simulink model "subsystem_socrates"  (R2019b)
settings: Solver=VariableStepAuto  StartTime=0.0  StopTime=10.0  RelTol=1e-3
undefined symbols (not defined in the file or in its folder): nb_rooms, nb_step_to_fifteen_min, nb_step_to_one_h, nb_step_to_thirty_min
libraries: dspstat3 x6
settings Model: Creator=guotong  LastModifiedBy=pat
settings ModelReferenceCC: ModelReferenceNumInstancesAllowed=Single

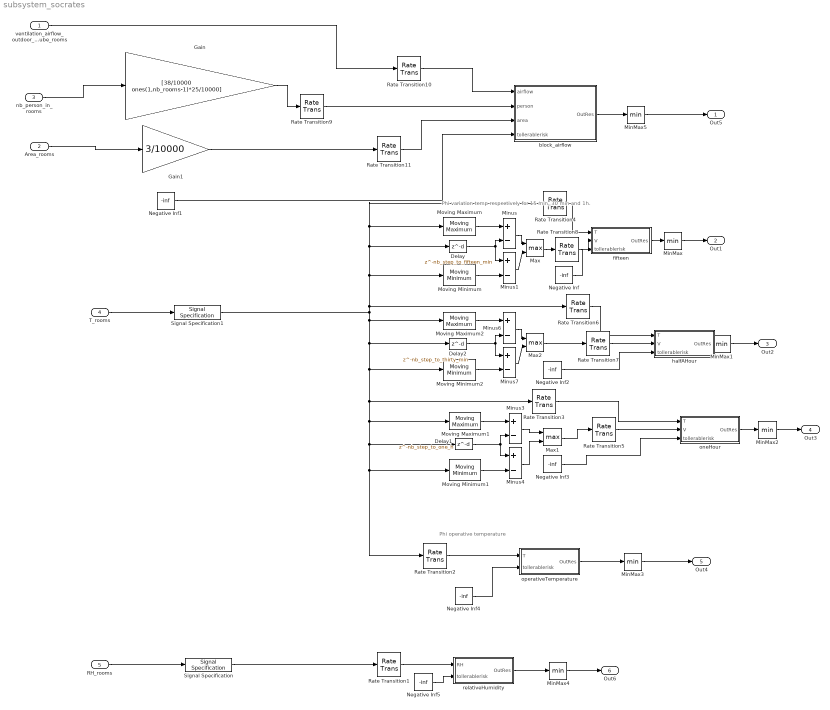
== system subsystem_socrates ==
  note: Phi operative temperature
  note: Phi variation temp respectively for 15 min, 30 min and 1h.
  ventilation_airflow_outdoor_air_mcube_rooms : Inport  PortDimensions=nb_rooms
  Area_rooms : Inport  Port=2  PortDimensions=nb_rooms
  nb_person_in_rooms : Inport  Port=3  OutDataTypeStr=double  PortDimensions=nb_rooms
  T_rooms : Inport  Port=4  PortDimensions=nb_rooms
  RH_rooms : Inport  Port=5  PortDimensions=nb_rooms
  Delay : Delay  DelayLength=nb_step_to_fifteen_min  InitialCondition=27
  Delay1 : Delay  DelayLength=nb_step_to_one_h  InitialCondition=27
  Delay2 : Delay  DelayLength=nb_step_to_thirty_min  InitialCondition=27
  Gain : Gain  Gain=[38/10000 ones(1,nb_rooms-1)*25/10000]
  Gain1 : Gain  Gain=3/10000
  Max : MinMax  Function=max  Inputs=2  ZeroCross=off
  Max1 : MinMax  Function=max  Inputs=2  ZeroCross=off
  Max2 : MinMax  Function=max  Inputs=2  ZeroCross=off
  MinMax{,1..5} (6 alike) : MinMax
  Minus{,1,3..4,6..7} (6 alike) : Sum  Inputs=+-
  Moving Maximum : dspstat3/Moving Maximum  SpecifyWindowLength=on  WindowLength=nb_step_to_fifteen_min  SimulateUsing=Code generation
      settings: SourceProductName=DSP System Toolbox  SourceProductBaseCode=DS
  Moving Maximum1 : dspstat3/Moving Maximum  SpecifyWindowLength=on  WindowLength=nb_step_to_one_h  SimulateUsing=Code generation
      settings: SourceProductName=DSP System Toolbox  SourceProductBaseCode=DS
  Moving Maximum2 : dspstat3/Moving Maximum  SpecifyWindowLength=on  WindowLength=nb_step_to_thirty_min  SimulateUsing=Code generation
      settings: SourceProductName=DSP System Toolbox  SourceProductBaseCode=DS
  Moving Minimum : dspstat3/Moving Minimum  SpecifyWindowLength=on  WindowLength=nb_step_to_fifteen_min  SimulateUsing=Code generation
      settings: SourceProductName=DSP System Toolbox  SourceProductBaseCode=DS
  Moving Minimum1 : dspstat3/Moving Minimum  SpecifyWindowLength=on  WindowLength=nb_step_to_one_h  SimulateUsing=Code generation
      settings: SourceProductName=DSP System Toolbox  SourceProductBaseCode=DS
  Moving Minimum2 : dspstat3/Moving Minimum  SpecifyWindowLength=on  WindowLength=nb_step_to_thirty_min  SimulateUsing=Code generation
      settings: SourceProductName=DSP System Toolbox  SourceProductBaseCode=DS
  Negative Inf{,1..5} (6 alike) : Constant  Value=-inf  OutDataTypeStr=Inherit: Inherit via back propagation
  Rate Transition{1..11} (11 alike) : RateTransition  OutPortSampleTime=rate
  Signal Specification : SignalSpecification  OutMin=-0.25  OutMax=1.25  Dimensions=nb_rooms
  Signal Specification1 : SignalSpecification  OutMin=-100  OutMax=100  Dimensions=nb_rooms
  block_airflow : Subsystem
  fifteen : Subsystem
  halfAHour : Subsystem
  oneHour : Subsystem
  operativeTemperature : Subsystem
  relativeHumidity : Subsystem
  Out5 : Outport
  Out1 : Outport  Port=2
  Out2 : Outport  Port=3
  Out3 : Outport  Port=4
  Out4 : Outport  Port=5
  Out6 : Outport  Port=6
  wires:
  nb_person_in_rooms/1 -> Gain/1
  Gain/1 -> Rate Transition9/1
  ventilation_airflow_outdoor_air_mcube_rooms/1 -> Rate Transition10/1
  Gain1/1 -> Rate Transition11/1
  Area_rooms/1 -> Gain1/1
  Delay2/1 -> Minus6/2, Minus7/1
  Moving Minimum1/1 -> Minus4/2
  Signal Specification1/1 -> Rate Transition2/1, Moving Minimum1/1, Delay1/1, Moving Maximum1/1, Rate Transition3/1, Moving Minimum2/1, Delay2/1, Moving Maximum2/1, Rate Transition6/1, Rate Transition4/1, Moving Maximum/1, Delay/1, Moving Minimum/1
  Delay/1 -> Minus1/1, Minus/2
  Moving Maximum/1 -> Minus/1
  Moving Maximum1/1 -> Minus3/1
  Moving Maximum2/1 -> Minus6/1
  Minus3/1 -> Max1/1
  Minus4/1 -> Max1/2
  Moving Minimum2/1 -> Minus7/2
  Delay1/1 -> Minus3/2, Minus4/1
  Minus1/1 -> Max/2
  Minus6/1 -> Max2/1
  Minus/1 -> Max/1
  Minus7/1 -> Max2/2
  Moving Minimum/1 -> Minus1/2
  T_rooms/1 -> Signal Specification1/1
  Signal Specification/1 -> Rate Transition1/1
  RH_rooms/1 -> Signal Specification/1
  Negative Inf4/1 -> operativeTemperature/2(tollerablerisk)
  Negative Inf2/1 -> halfAHour/3(tollerablerisk)
  Negative Inf/1 -> fifteen/3(tollerablerisk)
  Negative Inf5/1 -> relativeHumidity/2(tollerablerisk)
  Negative Inf1/1 -> block_airflow/4(tollerablerisk)
  block_airflow/1(OutRes) -> MinMax5/1
  fifteen/1(OutRes) -> MinMax/1
  halfAHour/1(OutRes) -> MinMax1/1
  oneHour/1(OutRes) -> MinMax2/1
  operativeTemperature/1(OutRes) -> MinMax3/1
  relativeHumidity/1(OutRes) -> MinMax4/1
  MinMax/1 -> Out1/1
  MinMax1/1 -> Out2/1
  MinMax2/1 -> Out3/1
  MinMax3/1 -> Out4/1
  MinMax4/1 -> Out6/1
  MinMax5/1 -> Out5/1
  Rate Transition1/1 -> relativeHumidity/1(RH)
  Rate Transition2/1 -> operativeTemperature/1(T)
  Rate Transition3/1 -> oneHour/1(T)
  Negative Inf3/1 -> oneHour/3(tollerablerisk)
  Max1/1 -> Rate Transition5/1
  Rate Transition5/1 -> oneHour/2(V)
  Rate Transition6/1 -> halfAHour/1(T)
  Rate Transition7/1 -> halfAHour/2(V)
  Max2/1 -> Rate Transition7/1
  Rate Transition4/1 -> fifteen/1(T)
  Max/1 -> Rate Transition8/1
  Rate Transition8/1 -> fifteen/2(V)
  Rate Transition9/1 -> block_airflow/2(person)
  Rate Transition10/1 -> block_airflow/1(airflow)
  Rate Transition11/1 -> block_airflow/3(area)

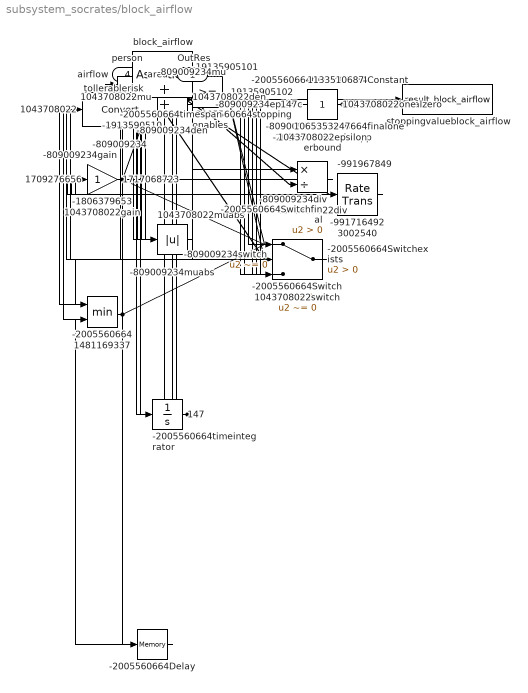
== system subsystem_socrates/block_airflow ==
  airflow : Inport
  person : Inport  Port=2
  area : Inport  Port=3
  tollerablerisk : Inport  Port=4
  -1806379653 : Gain
  -1913590510 : Logic  AllPortsSameDT=off  OutDataTypeStr=boolean
  -19135905101 : RelationalOperator  Operator=<=  OutDataTypeStr=boolean  RndMeth=Simplest
  -19135905102 : RelationalOperator  Operator=<=  OutDataTypeStr=boolean  RndMeth=Simplest
  -2005560664 : MinMax  Inputs=2
  -2005560664Constant : Constant
  -2005560664Delay : Memory  InitialCondition=1
  -2005560664Switch : Switch  Criteria=u2 > Threshold
  -2005560664Switchexists : Switch  Criteria=u2 > Threshold
  -2005560664Switchfinal : Switch  Criteria=u2 > Threshold
  -2005560664existupperbound : Constant  Value=0.0
  -2005560664finalone : Constant
  -2005560664finalzero : Constant  Value=0
  -2005560664stoppingenables : RelationalOperator  OutDataTypeStr=boolean  RndMeth=Simplest
  -2005560664timec : Constant
  -2005560664timeintegrator : Integrator
  -2005560664timespan : RelationalOperator  OutDataTypeStr=boolean  RndMeth=Simplest
  -809009234 : DataTypeConversion
  -809009234den : Sum
  -809009234div : Product  Inputs=*/
  -809009234epsilon : Constant  Value=-0.01
  -809009234gain : Gain
  -809009234mu : Sum  Inputs=+-
  -809009234muabs : Abs
  -809009234one : Constant
  -809009234switch : Switch  Criteria=u2 ~= 0
  -991716492 : RateTransition
  -991967849 : RateTransition
  1043708022 : DataTypeConversion
  1043708022den : Sum
  1043708022div : Product  Inputs=*/
  1043708022epsilon : Constant  Value=-0.01
  1043708022gain : Gain
  1043708022mu : Sum  Inputs=+-
  1043708022muabs : Abs
  1043708022one : Constant
  1043708022switch : Switch  Criteria=u2 ~= 0
  1065353247 : Constant  Value=1.0
  1133510687 : Constant  Value=288.0
  147 : Integrator
  147c : Constant
  1481169337 : MinMax  Inputs=2
  1709276656 : Gain
  1717068723 : Gain
  3002540 : RateTransition
  block_airflow : Assertion
  stoppingvalueblock_airflow : ToWorkspace  VariableName=result_block_airflow  SaveFormat=Timeseries  SampleTime=-1
      settings: MaxDataPoints=1
  OutRes : Outport
  wires:
  147c/1 -> 147/1
  1065353247/1 -> -19135905101/1
  147/1 -> -19135905101/2, -19135905102/1
  1133510687/1 -> -19135905102/2
  -19135905101/1 -> -1913590510/1
  -19135905102/1 -> -1913590510/2
  airflow/1 -> -991967849/1
  -991967849/1 -> 1709276656/1
  person/1 -> -991716492/1
  -991716492/1 -> 1717068723/1
  1709276656/1 -> 1043708022mu/1, -809009234mu/1
  1717068723/1 -> 1043708022mu/2
  1043708022mu/1 -> 1043708022muabs/1, 1043708022div/1, 1043708022switch/2
  1043708022muabs/1 -> 1043708022den/1
  1043708022one/1 -> 1043708022den/2
  1043708022den/1 -> 1043708022div/2
  1043708022div/1 -> 1043708022gain/1
  1043708022gain/1 -> 1043708022switch/1
  1043708022epsilon/1 -> 1043708022switch/3
  1043708022switch/1 -> 1043708022/1
  area/1 -> 3002540/1
  3002540/1 -> -1806379653/1
  -1806379653/1 -> -809009234mu/2
  -809009234mu/1 -> -809009234muabs/1, -809009234div/1, -809009234switch/2
  -809009234muabs/1 -> -809009234den/1
  -809009234one/1 -> -809009234den/2
  -809009234den/1 -> -809009234div/2
  -809009234div/1 -> -809009234gain/1
  -809009234gain/1 -> -809009234switch/1
  -809009234epsilon/1 -> -809009234switch/3
  -809009234switch/1 -> -809009234/1
  1043708022/1 -> 1481169337/2
  -809009234/1 -> 1481169337/1
  -2005560664Constant/1 -> -2005560664Switch/3
  -1913590510/1 -> -2005560664Switch/2
  1481169337/1 -> -2005560664Switch/1
  -2005560664Switch/1 -> -2005560664/1
  -2005560664/1 -> -2005560664Delay/1, OutRes/1, -2005560664timespan/2, stoppingvalueblock_airflow/1
  -2005560664Delay/1 -> -2005560664/2
  tollerablerisk/1 -> -2005560664timespan/1
  -2005560664finalzero/1 -> -2005560664Switchfinal/1, -2005560664Switchexists/3
  -2005560664timec/1 -> -2005560664timeintegrator/1
  -2005560664timeintegrator/1 -> -2005560664stoppingenables/1
  -2005560664existupperbound/1 -> -2005560664stoppingenables/2
  -2005560664stoppingenables/1 -> -2005560664Switchexists/2
  -2005560664timespan/1 -> -2005560664Switchexists/1
  -2005560664finalone/1 -> -2005560664Switchfinal/3
  -2005560664Switchexists/1 -> -2005560664Switchfinal/2
  -2005560664Switchfinal/1 -> block_airflow/1

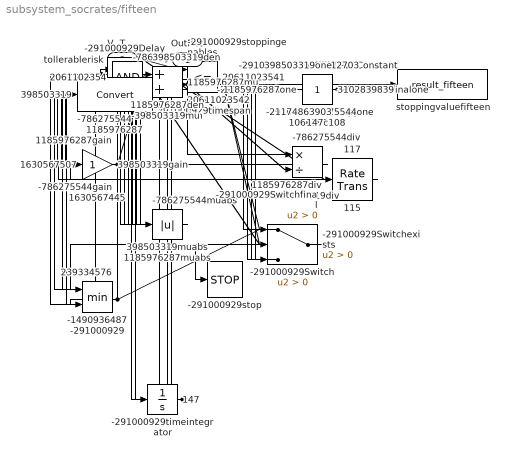
== system subsystem_socrates/fifteen ==
  T : Inport
  V : Inport  Port=2
  tollerablerisk : Inport  Port=3
  -1490936487 : MinMax  Function=max  Inputs=2
  -291000929 : MinMax  Inputs=2
  -291000929Constant : Constant
  -291000929Delay : UnitDelay  InitialCondition=1  SampleTime=-1  HasFrameUpgradeWarning=on
  -291000929Switch : Switch  Criteria=u2 > Threshold
  -291000929Switchexists : Switch  Criteria=u2 > Threshold
  -291000929Switchfinal : Switch  Criteria=u2 > Threshold
  -291000929existupperbound : Constant  Value=0.0
  -291000929finalone : Constant
  -291000929finalzero : Constant  Value=0
  -291000929stop : Stop
  -291000929stoppingenables : RelationalOperator  OutDataTypeStr=boolean  RndMeth=Simplest
  -291000929timec : Constant
  -291000929timeintegrator : Integrator
  -291000929timespan : RelationalOperator  OutDataTypeStr=boolean  RndMeth=Simplest
  -786275544 : DataTypeConversion
  -786275544den : Sum
  -786275544div : Product  Inputs=*/
  -786275544gain : Gain
  -786275544mu : Sum  Inputs=+-
  -786275544muabs : Abs
  -786275544one : Constant
  1066192108 : Constant  Value=1.1
  1102839839 : Constant  Value=23.5
  1104412703 : Constant  Value=26.5
  115 : RateTransition
  117 : RateTransition
  1174863903 : Constant  Value=8640.0
  1185976287 : DataTypeConversion
  1185976287den : Sum
  1185976287div : Product  Inputs=*/
  1185976287gain : Gain  Gain=-1
  1185976287mu : Sum  Inputs=+-
  1185976287muabs : Abs
  1185976287one : Constant
  147 : Integrator
  147c : Constant
  1630567445 : Gain
  1630567507 : Gain
  2061102354 : Logic  AllPortsSameDT=off  OutDataTypeStr=boolean
  20611023541 : RelationalOperator  Operator=<=  OutDataTypeStr=boolean  RndMeth=Simplest
  20611023542 : RelationalOperator  Operator=<=  OutDataTypeStr=boolean  RndMeth=Simplest
  239334576 : MinMax  Inputs=2
  31 : Constant  Value=0.0
  398503319 : DataTypeConversion
  398503319den : Sum
  398503319div : Product  Inputs=*/
  398503319gain : Gain
  398503319mu : Sum  Inputs=+-
  398503319muabs : Abs
  398503319one : Constant
  stoppingvaluefifteen : ToWorkspace  VariableName=result_fifteen  SaveFormat=Timeseries  SampleTime=-1
      settings: MaxDataPoints=1
  OutRes : Outport
  wires:
  147c/1 -> 147/1
  31/1 -> 20611023541/1
  147/1 -> 20611023541/2, 20611023542/1
  1174863903/1 -> 20611023542/2
  20611023541/1 -> 2061102354/1
  20611023542/1 -> 2061102354/2
  T/1 -> 115/1
  115/1 -> 1630567445/1
  1630567445/1 -> 1185976287mu/1, 398503319mu/1
  1102839839/1 -> 1185976287mu/2
  1185976287mu/1 -> 1185976287muabs/1, 1185976287div/1
  1185976287muabs/1 -> 1185976287den/1
  1185976287one/1 -> 1185976287den/2
  1185976287den/1 -> 1185976287div/2
  1185976287div/1 -> 1185976287gain/1
  1185976287gain/1 -> 1185976287/1
  1104412703/1 -> 398503319mu/2
  398503319mu/1 -> 398503319muabs/1, 398503319div/1
  398503319muabs/1 -> 398503319den/1
  398503319one/1 -> 398503319den/2
  398503319den/1 -> 398503319div/2
  398503319div/1 -> 398503319gain/1
  398503319gain/1 -> 398503319/1
  1185976287/1 -> -1490936487/2
  398503319/1 -> -1490936487/1
  V/1 -> 117/1
  117/1 -> 1630567507/1
  1630567507/1 -> -786275544mu/1
  1066192108/1 -> -786275544mu/2
  -786275544mu/1 -> -786275544muabs/1, -786275544div/1
  -786275544muabs/1 -> -786275544den/1
  -786275544one/1 -> -786275544den/2
  -786275544den/1 -> -786275544div/2
  -786275544div/1 -> -786275544gain/1
  -786275544gain/1 -> -786275544/1
  -1490936487/1 -> 239334576/2
  -786275544/1 -> 239334576/1
  -291000929Constant/1 -> -291000929Switch/3
  2061102354/1 -> -291000929Switch/2
  239334576/1 -> -291000929Switch/1
  -291000929Switch/1 -> -291000929/1
  -291000929/1 -> -291000929Delay/1, OutRes/1, -291000929timespan/2, stoppingvaluefifteen/1
  -291000929Delay/1 -> -291000929/2
  tollerablerisk/1 -> -291000929timespan/1
  -291000929finalzero/1 -> -291000929Switchfinal/3, -291000929Switchexists/3
  -291000929timec/1 -> -291000929timeintegrator/1
  -291000929timeintegrator/1 -> -291000929stoppingenables/1
  -291000929existupperbound/1 -> -291000929stoppingenables/2
  -291000929stoppingenables/1 -> -291000929Switchexists/2
  -291000929timespan/1 -> -291000929Switchexists/1
  -291000929finalone/1 -> -291000929Switchfinal/1
  -291000929Switchexists/1 -> -291000929Switchfinal/2
  -291000929Switchfinal/1 -> -291000929stop/1

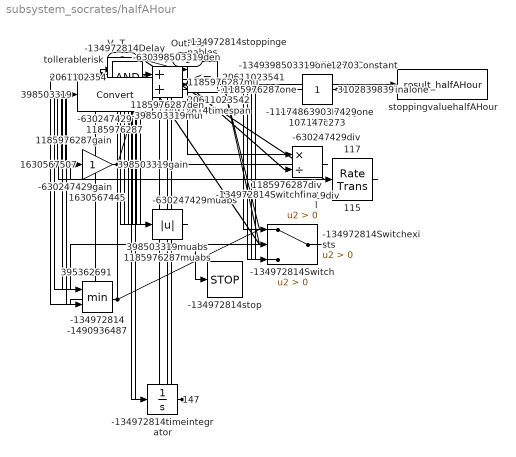
== system subsystem_socrates/halfAHour ==
  T : Inport
  V : Inport  Port=2
  tollerablerisk : Inport  Port=3
  -134972814 : MinMax  Inputs=2
  -134972814Constant : Constant
  -134972814Delay : UnitDelay  InitialCondition=1  SampleTime=-1  HasFrameUpgradeWarning=on
  -134972814Switch : Switch  Criteria=u2 > Threshold
  -134972814Switchexists : Switch  Criteria=u2 > Threshold
  -134972814Switchfinal : Switch  Criteria=u2 > Threshold
  -134972814existupperbound : Constant  Value=0.0
  -134972814finalone : Constant
  -134972814finalzero : Constant  Value=0
  -134972814stop : Stop
  -134972814stoppingenables : RelationalOperator  OutDataTypeStr=boolean  RndMeth=Simplest
  -134972814timec : Constant
  -134972814timeintegrator : Integrator
  -134972814timespan : RelationalOperator  OutDataTypeStr=boolean  RndMeth=Simplest
  -1490936487 : MinMax  Function=max  Inputs=2
  -630247429 : DataTypeConversion
  -630247429den : Sum
  -630247429div : Product  Inputs=*/
  -630247429gain : Gain
  -630247429mu : Sum  Inputs=+-
  -630247429muabs : Abs
  -630247429one : Constant
  1071225273 : Constant  Value=1.7
  1102839839 : Constant  Value=23.5
  1104412703 : Constant  Value=26.5
  115 : RateTransition
  117 : RateTransition
  1174863903 : Constant  Value=8640.0
  1185976287 : DataTypeConversion
  1185976287den : Sum
  1185976287div : Product  Inputs=*/
  1185976287gain : Gain  Gain=-1
  1185976287mu : Sum  Inputs=+-
  1185976287muabs : Abs
  1185976287one : Constant
  147 : Integrator
  147c : Constant
  1630567445 : Gain
  1630567507 : Gain
  2061102354 : Logic  AllPortsSameDT=off  OutDataTypeStr=boolean
  20611023541 : RelationalOperator  Operator=<=  OutDataTypeStr=boolean  RndMeth=Simplest
  20611023542 : RelationalOperator  Operator=<=  OutDataTypeStr=boolean  RndMeth=Simplest
  31 : Constant  Value=0.0
  395362691 : MinMax  Inputs=2
  398503319 : DataTypeConversion
  398503319den : Sum
  398503319div : Product  Inputs=*/
  398503319gain : Gain
  398503319mu : Sum  Inputs=+-
  398503319muabs : Abs
  398503319one : Constant
  stoppingvaluehalfAHour : ToWorkspace  VariableName=result_halfAHour  SaveFormat=Timeseries  SampleTime=-1
      settings: MaxDataPoints=1
  OutRes : Outport
  wires:
  147c/1 -> 147/1
  31/1 -> 20611023541/1
  147/1 -> 20611023541/2, 20611023542/1
  1174863903/1 -> 20611023542/2
  20611023541/1 -> 2061102354/1
  20611023542/1 -> 2061102354/2
  T/1 -> 115/1
  115/1 -> 1630567445/1
  1630567445/1 -> 1185976287mu/1, 398503319mu/1
  1102839839/1 -> 1185976287mu/2
  1185976287mu/1 -> 1185976287muabs/1, 1185976287div/1
  1185976287muabs/1 -> 1185976287den/1
  1185976287one/1 -> 1185976287den/2
  1185976287den/1 -> 1185976287div/2
  1185976287div/1 -> 1185976287gain/1
  1185976287gain/1 -> 1185976287/1
  1104412703/1 -> 398503319mu/2
  398503319mu/1 -> 398503319muabs/1, 398503319div/1
  398503319muabs/1 -> 398503319den/1
  398503319one/1 -> 398503319den/2
  398503319den/1 -> 398503319div/2
  398503319div/1 -> 398503319gain/1
  398503319gain/1 -> 398503319/1
  1185976287/1 -> -1490936487/2
  398503319/1 -> -1490936487/1
  V/1 -> 117/1
  117/1 -> 1630567507/1
  1630567507/1 -> -630247429mu/1
  1071225273/1 -> -630247429mu/2
  -630247429mu/1 -> -630247429muabs/1, -630247429div/1
  -630247429muabs/1 -> -630247429den/1
  -630247429one/1 -> -630247429den/2
  -630247429den/1 -> -630247429div/2
  -630247429div/1 -> -630247429gain/1
  -630247429gain/1 -> -630247429/1
  -1490936487/1 -> 395362691/2
  -630247429/1 -> 395362691/1
  -134972814Constant/1 -> -134972814Switch/3
  2061102354/1 -> -134972814Switch/2
  395362691/1 -> -134972814Switch/1
  -134972814Switch/1 -> -134972814/1
  -134972814/1 -> -134972814Delay/1, OutRes/1, -134972814timespan/2, stoppingvaluehalfAHour/1
  -134972814Delay/1 -> -134972814/2
  tollerablerisk/1 -> -134972814timespan/1
  -134972814finalzero/1 -> -134972814Switchfinal/3, -134972814Switchexists/3
  -134972814timec/1 -> -134972814timeintegrator/1
  -134972814timeintegrator/1 -> -134972814stoppingenables/1
  -134972814existupperbound/1 -> -134972814stoppingenables/2
  -134972814stoppingenables/1 -> -134972814Switchexists/2
  -134972814timespan/1 -> -134972814Switchexists/1
  -134972814finalone/1 -> -134972814Switchfinal/1
  -134972814Switchexists/1 -> -134972814Switchfinal/2
  -134972814Switchfinal/1 -> -134972814stop/1

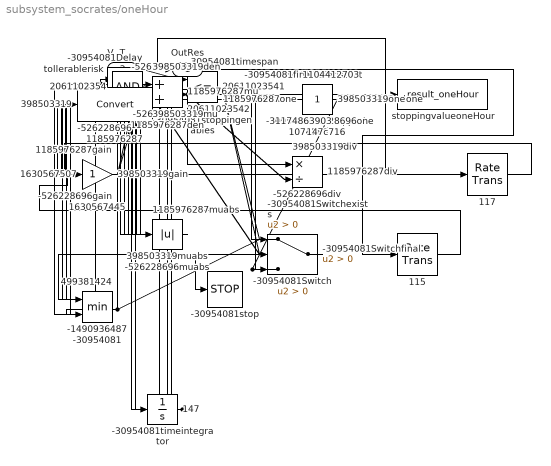
== system subsystem_socrates/oneHour ==
  T : Inport
  V : Inport  Port=2
  tollerablerisk : Inport  Port=3
  -1490936487 : MinMax  Function=max  Inputs=2
  -30954081 : MinMax  Inputs=2
  -30954081Constant : Constant
  -30954081Delay : UnitDelay  InitialCondition=1  SampleTime=-1  HasFrameUpgradeWarning=on
  -30954081Switch : Switch  Criteria=u2 > Threshold
  -30954081Switchexists : Switch  Criteria=u2 > Threshold
  -30954081Switchfinal : Switch  Criteria=u2 > Threshold
  -30954081existupperbound : Constant  Value=0.0
  -30954081finalone : Constant
  -30954081finalzero : Constant  Value=0
  -30954081stop : Stop
  -30954081stoppingenables : RelationalOperator  OutDataTypeStr=boolean  RndMeth=Simplest
  -30954081timec : Constant
  -30954081timeintegrator : Integrator
  -30954081timespan : RelationalOperator  OutDataTypeStr=boolean  RndMeth=Simplest
  -526228696 : DataTypeConversion
  -526228696den : Sum
  -526228696div : Product  Inputs=*/
  -526228696gain : Gain
  -526228696mu : Sum  Inputs=+-
  -526228696muabs : Abs
  -526228696one : Constant
  1074580716 : Constant  Value=2.2
  1102839839 : Constant  Value=23.5
  1104412703 : Constant  Value=26.5
  115 : RateTransition
  117 : RateTransition
  1174863903 : Constant  Value=8640.0
  1185976287 : DataTypeConversion
  1185976287den : Sum
  1185976287div : Product  Inputs=*/
  1185976287gain : Gain  Gain=-1
  1185976287mu : Sum  Inputs=+-
  1185976287muabs : Abs
  1185976287one : Constant
  147 : Integrator
  147c : Constant
  1630567445 : Gain
  1630567507 : Gain
  2061102354 : Logic  AllPortsSameDT=off  OutDataTypeStr=boolean
  20611023541 : RelationalOperator  Operator=<=  OutDataTypeStr=boolean  RndMeth=Simplest
  20611023542 : RelationalOperator  Operator=<=  OutDataTypeStr=boolean  RndMeth=Simplest
  31 : Constant  Value=0.0
  398503319 : DataTypeConversion
  398503319den : Sum
  398503319div : Product  Inputs=*/
  398503319gain : Gain
  398503319mu : Sum  Inputs=+-
  398503319muabs : Abs
  398503319one : Constant
  499381424 : MinMax  Inputs=2
  stoppingvalueoneHour : ToWorkspace  VariableName=result_oneHour  SaveFormat=Timeseries  SampleTime=-1
      settings: MaxDataPoints=1
  OutRes : Outport
  wires:
  147c/1 -> 147/1
  31/1 -> 20611023541/1
  147/1 -> 20611023541/2, 20611023542/1
  1174863903/1 -> 20611023542/2
  20611023541/1 -> 2061102354/1
  20611023542/1 -> 2061102354/2
  T/1 -> 115/1
  115/1 -> 1630567445/1
  1630567445/1 -> 1185976287mu/1, 398503319mu/1
  1102839839/1 -> 1185976287mu/2
  1185976287mu/1 -> 1185976287muabs/1, 1185976287div/1
  1185976287muabs/1 -> 1185976287den/1
  1185976287one/1 -> 1185976287den/2
  1185976287den/1 -> 1185976287div/2
  1185976287div/1 -> 1185976287gain/1
  1185976287gain/1 -> 1185976287/1
  1104412703/1 -> 398503319mu/2
  398503319mu/1 -> 398503319muabs/1, 398503319div/1
  398503319muabs/1 -> 398503319den/1
  398503319one/1 -> 398503319den/2
  398503319den/1 -> 398503319div/2
  398503319div/1 -> 398503319gain/1
  398503319gain/1 -> 398503319/1
  1185976287/1 -> -1490936487/2
  398503319/1 -> -1490936487/1
  V/1 -> 117/1
  117/1 -> 1630567507/1
  1630567507/1 -> -526228696mu/1
  1074580716/1 -> -526228696mu/2
  -526228696mu/1 -> -526228696muabs/1, -526228696div/1
  -526228696muabs/1 -> -526228696den/1
  -526228696one/1 -> -526228696den/2
  -526228696den/1 -> -526228696div/2
  -526228696div/1 -> -526228696gain/1
  -526228696gain/1 -> -526228696/1
  -1490936487/1 -> 499381424/2
  -526228696/1 -> 499381424/1
  -30954081Constant/1 -> -30954081Switch/3
  2061102354/1 -> -30954081Switch/2
  499381424/1 -> -30954081Switch/1
  -30954081Switch/1 -> -30954081/1
  -30954081/1 -> -30954081Delay/1, OutRes/1, -30954081timespan/2, stoppingvalueoneHour/1
  -30954081Delay/1 -> -30954081/2
  tollerablerisk/1 -> -30954081timespan/1
  -30954081finalzero/1 -> -30954081Switchfinal/3, -30954081Switchexists/3
  -30954081timec/1 -> -30954081timeintegrator/1
  -30954081timeintegrator/1 -> -30954081stoppingenables/1
  -30954081existupperbound/1 -> -30954081stoppingenables/2
  -30954081stoppingenables/1 -> -30954081Switchexists/2
  -30954081timespan/1 -> -30954081Switchexists/1
  -30954081finalone/1 -> -30954081Switchfinal/1
  -30954081Switchexists/1 -> -30954081Switchfinal/2
  -30954081Switchfinal/1 -> -30954081stop/1

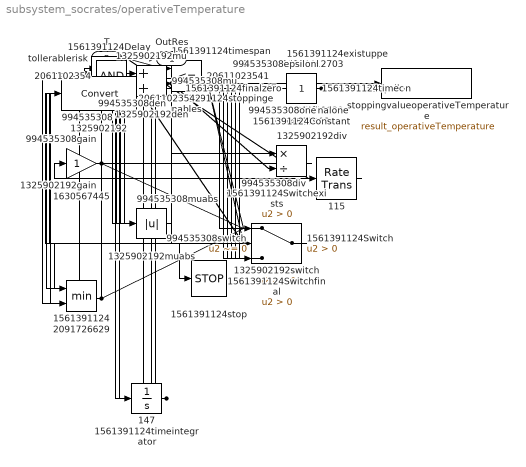
== system subsystem_socrates/operativeTemperature ==
  T : Inport
  tollerablerisk : Inport  Port=2
  1102839839 : Constant  Value=23.5
  1104412703 : Constant  Value=26.5
  115 : RateTransition
  1174863903 : Constant  Value=8640.0
  1325902192 : DataTypeConversion
  1325902192den : Sum
  1325902192div : Product  Inputs=*/
  1325902192epsilon : Constant  Value=-0.01
  1325902192gain : Gain  Gain=-1
  1325902192mu : Sum  Inputs=+-
  1325902192muabs : Abs
  1325902192one : Constant
  1325902192switch : Switch  Criteria=u2 ~= 0
  147 : Integrator
  147c : Constant
  1561391124 : MinMax  Inputs=2
  1561391124Constant : Constant
  1561391124Delay : UnitDelay  InitialCondition=1  SampleTime=-1  HasFrameUpgradeWarning=on
  1561391124Switch : Switch  Criteria=u2 > Threshold
  1561391124Switchexists : Switch  Criteria=u2 > Threshold
  1561391124Switchfinal : Switch  Criteria=u2 > Threshold
  1561391124existupperbound : Constant  Value=0.0
  1561391124finalone : Constant
  1561391124finalzero : Constant  Value=0
  1561391124stop : Stop
  1561391124stoppingenables : RelationalOperator  OutDataTypeStr=boolean  RndMeth=Simplest
  1561391124timec : Constant
  1561391124timeintegrator : Integrator
  1561391124timespan : RelationalOperator  OutDataTypeStr=boolean  RndMeth=Simplest
  1630567445 : Gain
  2061102354 : Logic  AllPortsSameDT=off  OutDataTypeStr=boolean
  20611023541 : RelationalOperator  Operator=<=  OutDataTypeStr=boolean  RndMeth=Simplest
  20611023542 : RelationalOperator  Operator=<=  OutDataTypeStr=boolean  RndMeth=Simplest
  2091726629 : MinMax  Inputs=2
  31 : Constant  Value=0.0
  994535308 : DataTypeConversion
  994535308den : Sum
  994535308div : Product  Inputs=*/
  994535308epsilon : Constant  Value=-0.01
  994535308gain : Gain
  994535308mu : Sum  Inputs=+-
  994535308muabs : Abs
  994535308one : Constant
  994535308switch : Switch  Criteria=u2 ~= 0
  stoppingvalueoperativeTemperature : ToWorkspace  VariableName=result_operativeTemperature  SaveFormat=Timeseries  SampleTime=-1
      settings: MaxDataPoints=1
  OutRes : Outport
  wires:
  147c/1 -> 147/1
  31/1 -> 20611023541/1
  147/1 -> 20611023541/2, 20611023542/1
  1174863903/1 -> 20611023542/2
  20611023541/1 -> 2061102354/1
  20611023542/1 -> 2061102354/2
  T/1 -> 115/1
  115/1 -> 1630567445/1
  1630567445/1 -> 994535308mu/1, 1325902192mu/1
  1102839839/1 -> 994535308mu/2
  994535308mu/1 -> 994535308muabs/1, 994535308div/1, 994535308switch/2
  994535308muabs/1 -> 994535308den/1
  994535308one/1 -> 994535308den/2
  994535308den/1 -> 994535308div/2
  994535308div/1 -> 994535308gain/1
  994535308gain/1 -> 994535308switch/1
  994535308epsilon/1 -> 994535308switch/3
  994535308switch/1 -> 994535308/1
  1104412703/1 -> 1325902192mu/2
  1325902192mu/1 -> 1325902192muabs/1, 1325902192div/1, 1325902192switch/2
  1325902192muabs/1 -> 1325902192den/1
  1325902192one/1 -> 1325902192den/2
  1325902192den/1 -> 1325902192div/2
  1325902192div/1 -> 1325902192gain/1
  1325902192gain/1 -> 1325902192switch/1
  1325902192epsilon/1 -> 1325902192switch/3
  1325902192switch/1 -> 1325902192/1
  994535308/1 -> 2091726629/2
  1325902192/1 -> 2091726629/1
  1561391124Constant/1 -> 1561391124Switch/3
  2061102354/1 -> 1561391124Switch/2
  2091726629/1 -> 1561391124Switch/1
  1561391124Switch/1 -> 1561391124/1
  1561391124/1 -> 1561391124Delay/1, OutRes/1, 1561391124timespan/2, stoppingvalueoperativeTemperature/1
  1561391124Delay/1 -> 1561391124/2
  tollerablerisk/1 -> 1561391124timespan/1
  1561391124finalzero/1 -> 1561391124Switchfinal/3, 1561391124Switchexists/3
  1561391124timec/1 -> 1561391124timeintegrator/1
  1561391124timeintegrator/1 -> 1561391124stoppingenables/1
  1561391124existupperbound/1 -> 1561391124stoppingenables/2
  1561391124stoppingenables/1 -> 1561391124Switchexists/2
  1561391124timespan/1 -> 1561391124Switchexists/1
  1561391124finalone/1 -> 1561391124Switchfinal/1
  1561391124Switchexists/1 -> 1561391124Switchfinal/2
  1561391124Switchfinal/1 -> 1561391124stop/1

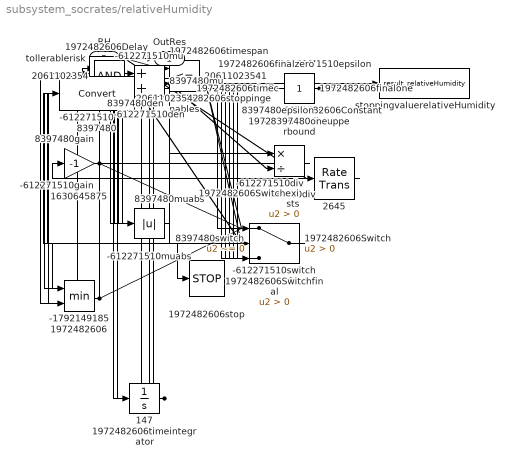
== system subsystem_socrates/relativeHumidity ==
  RH : Inport
  tollerablerisk : Inport  Port=2
  -1792149185 : MinMax  Inputs=2
  -612271510 : DataTypeConversion
  -612271510den : Sum
  -612271510div : Product  Inputs=*/
  -612271510epsilon : Constant  Value=-0.01
  -612271510gain : Gain
  -612271510mu : Sum  Inputs=+-
  -612271510muabs : Abs
  -612271510one : Constant
  -612271510switch : Switch  Criteria=u2 ~= 0
  1048576031 : Constant  Value=0.25
  1059481221 : Constant  Value=0.65
  1174863903 : Constant  Value=8640.0
  147 : Integrator
  147c : Constant
  1630645875 : Gain
  1972482606 : MinMax  Inputs=2
  1972482606Constant : Constant
  1972482606Delay : UnitDelay  InitialCondition=1  SampleTime=-1  HasFrameUpgradeWarning=on
  1972482606Switch : Switch  Criteria=u2 > Threshold
  1972482606Switchexists : Switch  Criteria=u2 > Threshold
  1972482606Switchfinal : Switch  Criteria=u2 > Threshold
  1972482606existupperbound : Constant  Value=0.0
  1972482606finalone : Constant
  1972482606finalzero : Constant  Value=0
  1972482606stop : Stop
  1972482606stoppingenables : RelationalOperator  OutDataTypeStr=boolean  RndMeth=Simplest
  1972482606timec : Constant
  1972482606timeintegrator : Integrator
  1972482606timespan : RelationalOperator  OutDataTypeStr=boolean  RndMeth=Simplest
  2061102354 : Logic  AllPortsSameDT=off  OutDataTypeStr=boolean
  20611023541 : RelationalOperator  Operator=<=  OutDataTypeStr=boolean  RndMeth=Simplest
  20611023542 : RelationalOperator  Operator=<=  OutDataTypeStr=boolean  RndMeth=Simplest
  2645 : RateTransition
  31 : Constant  Value=0.0
  8397480 : DataTypeConversion
  8397480den : Sum
  8397480div : Product  Inputs=*/
  8397480epsilon : Constant  Value=-0.01
  8397480gain : Gain  Gain=-1
  8397480mu : Sum  Inputs=+-
  8397480muabs : Abs
  8397480one : Constant
  8397480switch : Switch  Criteria=u2 ~= 0
  stoppingvaluerelativeHumidity : ToWorkspace  VariableName=result_relativeHumidity  SaveFormat=Timeseries  SampleTime=-1
      settings: MaxDataPoints=1
  OutRes : Outport
  wires:
  147c/1 -> 147/1
  31/1 -> 20611023541/1
  147/1 -> 20611023541/2, 20611023542/1
  1174863903/1 -> 20611023542/2
  20611023541/1 -> 2061102354/1
  20611023542/1 -> 2061102354/2
  RH/1 -> 2645/1
  2645/1 -> 1630645875/1
  1630645875/1 -> -612271510mu/1, 8397480mu/1
  1048576031/1 -> -612271510mu/2
  -612271510mu/1 -> -612271510muabs/1, -612271510div/1, -612271510switch/2
  -612271510muabs/1 -> -612271510den/1
  -612271510one/1 -> -612271510den/2
  -612271510den/1 -> -612271510div/2
  -612271510div/1 -> -612271510gain/1
  -612271510gain/1 -> -612271510switch/1
  -612271510epsilon/1 -> -612271510switch/3
  -612271510switch/1 -> -612271510/1
  1059481221/1 -> 8397480mu/2
  8397480mu/1 -> 8397480muabs/1, 8397480div/1, 8397480switch/2
  8397480muabs/1 -> 8397480den/1
  8397480one/1 -> 8397480den/2
  8397480den/1 -> 8397480div/2
  8397480div/1 -> 8397480gain/1
  8397480gain/1 -> 8397480switch/1
  8397480epsilon/1 -> 8397480switch/3
  8397480switch/1 -> 8397480/1
  -612271510/1 -> -1792149185/2
  8397480/1 -> -1792149185/1
  1972482606Constant/1 -> 1972482606Switch/3
  2061102354/1 -> 1972482606Switch/2
  -1792149185/1 -> 1972482606Switch/1
  1972482606Switch/1 -> 1972482606/1
  1972482606/1 -> 1972482606Delay/1, OutRes/1, 1972482606timespan/2, stoppingvaluerelativeHumidity/1
  1972482606Delay/1 -> 1972482606/2
  tollerablerisk/1 -> 1972482606timespan/1
  1972482606finalzero/1 -> 1972482606Switchfinal/3, 1972482606Switchexists/3
  1972482606timec/1 -> 1972482606timeintegrator/1
  1972482606timeintegrator/1 -> 1972482606stoppingenables/1
  1972482606existupperbound/1 -> 1972482606stoppingenables/2
  1972482606stoppingenables/1 -> 1972482606Switchexists/2
  1972482606timespan/1 -> 1972482606Switchexists/1
  1972482606finalone/1 -> 1972482606Switchfinal/1
  1972482606Switchexists/1 -> 1972482606Switchfinal/2
  1972482606Switchfinal/1 -> 1972482606stop/1
